simulink model "rtwdemo_forloop"  (Simulink 6.0)
settings: Solver=ode5  StartTime=0.0  StopTime=10.0  RelTol=1e-3
libraries: rtwdemowidgets x2
settings Model: Creator=The MathWorks Inc.  LastModifiedBy=batserve  ExtModeAutoUpdateStatusClock=off
settings DataIOCC: SaveFormat=StructureWithTime  SaveOutput=off  SaveTime=off  SignalLoggingName=sigsOut
settings OptimizationCC: InlineParams=on  EnforceIntegerDowncast=off  StateBitsets=on  DataBitsets=on  UseTempVars=on
settings DebuggingCC: CheckExecutionContextPreStartOutputMsg=on  CheckExecutionContextRuntimeOutputMsg=on  SolverPrmCheckMsg=none
settings RTWCC: TLCOptions=-p0 -aWarnNonSaturatedBlocks=0  GenerateReport=on  RTWVerbose=off  ProcessScript=grt_make_rtw_hook  LaunchReport=on
settings CodeAppCC: ForceParamTrailComments=on
settings GRTTargetCC: MatFileLogging=off

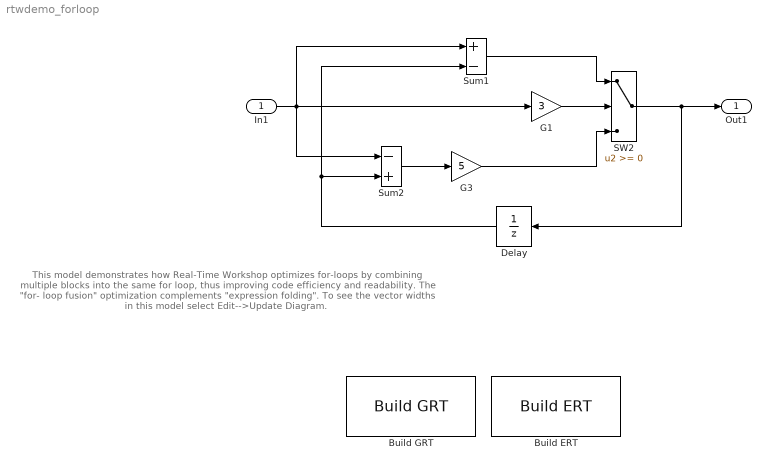
== system rtwdemo_forloop ==
  note: This model demonstrates how Real-Time Workshop optimizes for-loops by combining multiple
      | blocks into the same for loop, thus improving code efficiency and readability.  The "for-
      | loop fusion" optimization complements "expression folding".  To see the vector widths
      | in this model select Edit-->Update Diagram.
  In1 : Inport  Port=1  PortDimensions=10  LatchInput=off
  Build ERT : rtwdemowidgets/Build ERT  attrib_overrides={}
  Build GRT : rtwdemowidgets/Build GRT  attrib_overrides={}
  Delay : UnitDelay  Orientation=left
  G1 : Gain  Gain=3  SaturateOnIntegerOverflow=on
  G3 : Gain  Gain=5  SaturateOnIntegerOverflow=on
  SW2 : Switch  ZeroCross=off  SaturateOnIntegerOverflow=on  InputSameDT=on
  Sum1 : Sum  Inputs=+-  SaturateOnIntegerOverflow=on  InputSameDT=on
  Sum2 : Sum  Inputs=-+  SaturateOnIntegerOverflow=on  InputSameDT=on
  Out1 : Outport
  wires:
  Sum1/1 -> SW2/1
  G1/1 -> SW2/2
  Sum2/1 -> G3/1
  SW2/1 -> Delay/1, Out1/1
  Delay/1 -> Sum2/2, Sum1/2
  In1/1 -> G1/1, Sum1/1, Sum2/1
  G3/1 -> SW2/3
